simulink model "fisher"  (R2014b)
settings: Solver=ode4  StartTime=0.0  StopTime=10  FixedStep=0.001  RelTol=1e-3
values from neighbouring files (symbols this model uses):
  n = input(prompt)    [init.m]    (also in init_consensus.m = 4; init_consensus_15.m = 15; init_mussels.m = 5; init_mussels_2.m = 5)
undefined symbols (not defined in the file or in its folder): X, Y
settings Model: Creator=Demijan  LastModifiedBy=Demijan
settings DebuggingCC: SignalResolutionControl=TryResolveAll

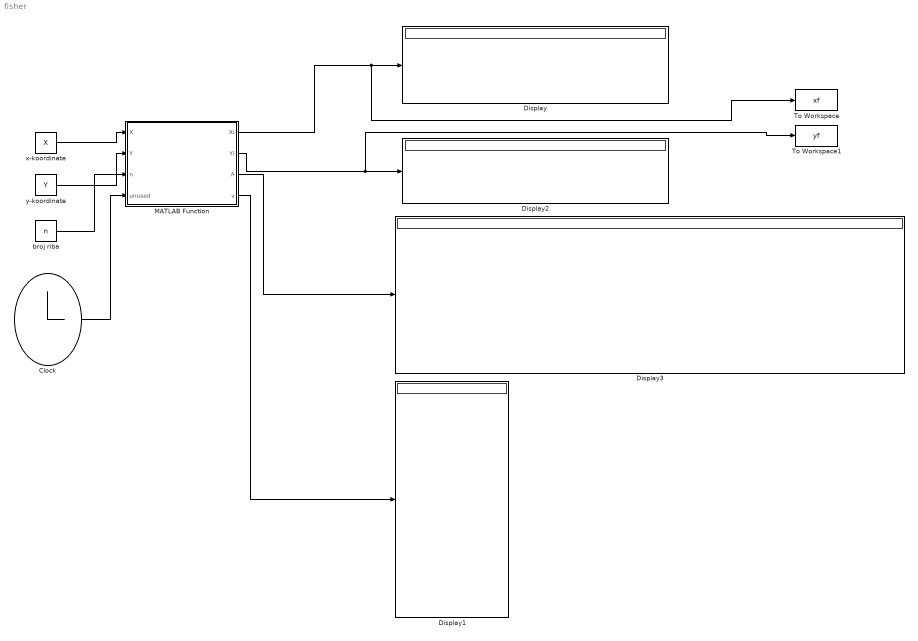
== system fisher ==
  Clock : Clock
  Display{,1..3} (4 alike) : Display
  MATLAB Function : MATLAB Function  TreatAsAtomicUnit=on
  To Workspace : ToWorkspace  VariableName=xf  SaveFormat=Structure  SampleTime=-1
  To Workspace1 : ToWorkspace  VariableName=yf  SaveFormat=Structure  SampleTime=-1
  broj riba : Constant  Value=n
  x-koordinate : Constant  Value=X
  y-koordinate : Constant  Value=Y
  wires:
  x-koordinate/1 -> MATLAB Function/1(X)
  MATLAB Function/1(Xi) -> To Workspace/1, Display/1
  MATLAB Function/2(Yi) -> To Workspace1/1, Display2/1
  y-koordinate/1 -> MATLAB Function/2(Y)
  broj riba/1 -> MATLAB Function/3(n)
  MATLAB Function/3(A) -> Display3/1
  MATLAB Function/4(v) -> Display1/1
  Clock/1 -> MATLAB Function/4(unused)

== matlab function fisher/MATLAB Function ==
  settings: updateMethod=DISCRETE  sampleTime=0.001
  data: X input; Xi output size=20 [0..20]; Yi output size=20 [0..20]; Y input; n input; A output; v output; unused input
function [Xi, Yi, A, v] = fish(X, Y, n, ~)

%#codegen
%zelim ovo samo prvi put(init??)
Xi=X;
Yi=Y;
A=zeros(10,10);
v=zeros(10,2);
%radius i brzine
for i=1:n;
    if rand >0.5;
    v(i,1)=-100*rand;
    v(i,2)=100*rand;
    else
    v(i,1)=100*rand;
    v(i,2)=-100*rand; 
    end
    for j=1:n;
        R = sqrt(((Xi(i)-Xi(j))^2+(Yi(i)-Yi(j))^2));
        if R < 4;
            A(i,j)=1;
        else
            A(i,j)=0;
        end
    end
end;
for i=1:n;
    Xi(i)=Xi(i)+0.001*v(i,1);
    Yi(i)=Yi(i)+0.001*v(i,2);
end;
end
